simulink model "mymodel"  (R2019b)
settings: Solver=VariableStepAuto  StartTime=0.0  StopTime=20  RelTol=1e-3
settings Model: Creator=mountj  LastModifiedBy=n9182250
settings DataIOCC: TimeSaveName=mytime

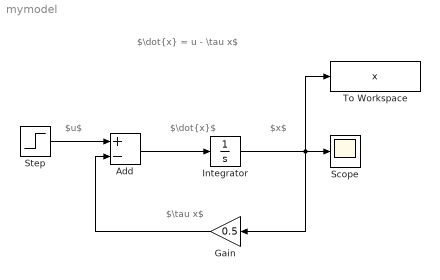
== system mymodel ==
  note: $\dot{x}$
  note: $x$
  note: $\dot{x} = u - \tau x$
  note: $u$
  note: $\tau x$
  Add : Sum  Inputs=+-
  Gain : Gain  Gain=0.5
  Integrator : Integrator
  Scope : Scope
  Step : Step  After=10  SampleTime=0
  To Workspace : ToWorkspace  VariableName=x  SampleTime=-1
  wires:
  Step/1 -> Add/1
  Add/1 -> Integrator/1
  Integrator/1 -> Gain/1, Scope/1, To Workspace/1
  Gain/1 -> Add/2
